simulink model "Observer_mode_model"  (R2023a)
settings: Solver=VariableStepAuto  StartTime=0.0  StopTime=10.0  RelTol=1e-3
settings Model: Creator=The MathWorks, Inc.  LastModifiedBy=bened
settings SolverCC: MaxZcPerStep=1
settings DebuggingCC: UnconnectedInputMsg=warning  UnconnectedOutputMsg=warning  UnconnectedLineMsg=warning
settings ModelReferenceCC: EnableRefExpFcnMdlSchedulingChecks=on
settings RTWCC: DLArmComputeVersion=19.05

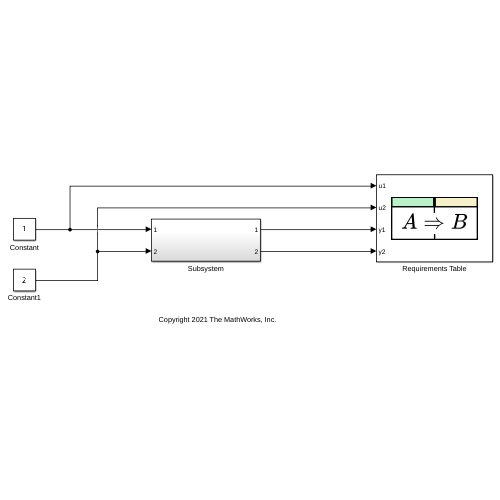
[thumbnail: Simulink's stored preview of the top-level diagram]
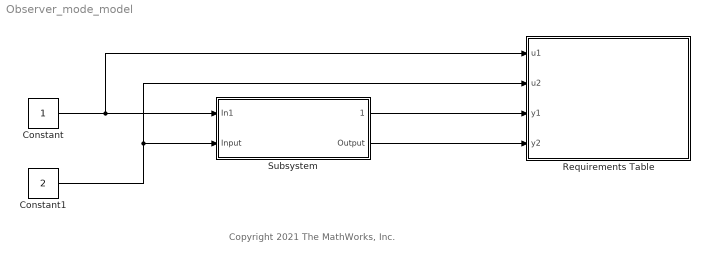
== system Observer_mode_model ==
  note: Copyright 2021 The MathWorks, Inc.
  Constant : Constant
  Constant1 : Constant  Value=2
  Requirements Table : Requirements Table  TreatAsAtomicUnit=on
  Subsystem : Subsystem
  wires:
  Subsystem/2(Output) -> Requirements Table/4(y2)
  Constant/1 -> Subsystem/1(In1), Requirements Table/1(u1)
  Constant1/1 -> Subsystem/2(Input), Requirements Table/2(u2)
  Subsystem/1(1) -> Requirements Table/3(y1)

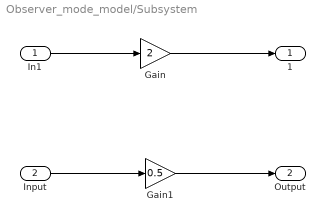
== system Observer_mode_model/Subsystem ==
  In1 : Inport
  Input : Inport  Port=2
  Gain : Gain  Gain=2
  Gain1 : Gain  Gain=0.5
  1 : Outport
  Output : Outport  Port=2
  wires:
  Gain/1 -> 1/1
  In1/1 -> Gain/1
  Input/1 -> Gain1/1
  Gain1/1 -> Output/1

== stateflow chart Observer_mode_model/Requirements Table ==
  (default) -> (junction 1073742737)
  (junction 1073742737) -> (junction 1073742738) : {
      | % SF_REQ_REV_07
      | }
  (junction 1073742738) -> (junction 1073742740) : {
      | % HEADER_ASSIGNMENTS
      |
      | }
  (junction 1073742740) -> (junction 1073742742) : {
      | % START_A_4
      | }
  (junction 1073742742) -> (junction 1073742744) : {
      | }
  (junction 1073742744) -> (junction 1073742746)
  (junction 1073742746) -> (junction 1073742748) : {
      | }
  (junction 1073742748) -> (junction 1073742750) : {
      | % END_A_4
      | }
  (junction 1073742750) -> (junction 1073742752) : {
      | % START_R_7
      | }
  (junction 1073742752) -> (junction 1073742754) : {
      | }
  (junction 1073742754) -> (junction 1073742756)
  (junction 1073742756) -> (junction 1073742758) [order 1] : [(u1 > 0)]
  (junction 1073742756) -> (junction 1073742764) [order 2]
  (junction 1073742758) -> (junction 1073742760) : {
      | reqtable_postcondition((y1 == 2), 'R:1');
      |
      |
      | }
  (junction 1073742760) -> (junction 1073742762) : {
      | }
  (junction 1073742762) -> (junction 1073742764)
  (junction 1073742764) -> (junction 1073742766)
  (junction 1073742766) -> (junction 1073742768) : {
      | % END_R_7
      | }
  (junction 1073742768) -> (junction 1073742770) : {
      | % START_R_1
      | }
  (junction 1073742770) -> (junction 1073742772) : {
      | }
  (junction 1073742772) -> (junction 1073742774)
  (junction 1073742774) -> (junction 1073742776) [order 1] : [(u2 > 0)]
  (junction 1073742774) -> (junction 1073742782) [order 2]
  (junction 1073742776) -> (junction 1073742778) : {
      | reqtable_postcondition((y2 > 0), 'R:2');
      |
      |
      | }
  (junction 1073742778) -> (junction 1073742780) : {
      | }
  (junction 1073742780) -> (junction 1073742782)
  (junction 1073742782) -> (junction 1073742784)
  (junction 1073742784) -> (junction 1073742786) : {
      | % END_R_1
      | }
  data: u1 input; u2 input; y1 input; y2 input
